simulink model "LKATestBenchExample"  (R2025b)
settings: Solver=VariableStepAuto  StartTime=0.0  StopTime=simStopTime  RelTol=1e-3
PostLoadFcn:
  | helperLKASetUp
StartFcn:
  | %sound(y_audio,Fs_audio);
values from neighbouring files (symbols this model uses):
  egoID = egoVehicle.ActorID    [helperLKASetUp.m]
  lr = 1.6    [helperLKASetUp.m]
  m = 1575    [helperLKASetUp.m]
  simStopTime = 30    [createDriverPath.m]
  Ts_3D = 0.1    [helperLKASetUp.m]
undefined symbols (not defined in the file or in its folder): Curvature, CurvatureDerivative, driving, gray, HeadingAngle, LateralOffset, Left, Right, Sim3dSensor, Strength, v0_ego, x0_ego, y0_ego, yaw0_ego
libraries: drivingscenarioandsensors x3, vrlib x1, sim3dcameralib x1, sim3dlib x1, sim3dautolib x1, dspvision x1, autolibshared x1
CloseFcn:
  | helperLKACleanUp
settings Model: SimulationMode=accelerator  Creator=The MathWorks, Inc.  LastModifiedBy=diogo
settings SolverCC: AlgebraicLoopSolver=TrustRegion
settings DataIOCC: ReturnWorkspaceOutputs=off
settings DebuggingCC: ParameterPrecisionLossMsg=none  UnconnectedInputMsg=warning  UnconnectedOutputMsg=warning  UnconnectedLineMsg=warning  ArithmeticOperatorsInVariantConditions=warning
settings HardwareCC: ProdLongLongMode=on
settings ModelReferenceCC: EnableRefExpFcnMdlSchedulingChecks=on
settings SFSimCC: SimUseLocalCustomCode=off
settings RTWCC: RTWUseLocalCustomCode=off  GPUComputeCapability=3.5  DLArmComputeVersion=19.05

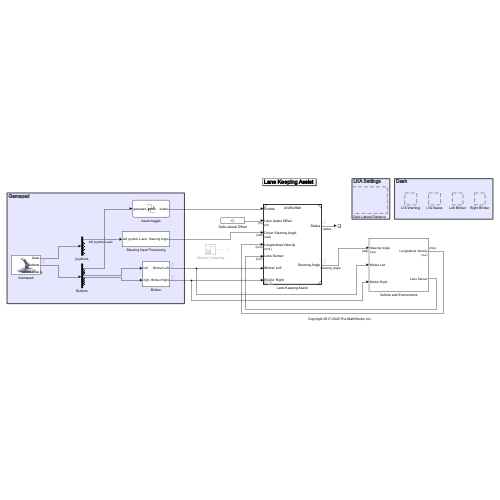
[thumbnail: Simulink's stored preview of the top-level diagram]
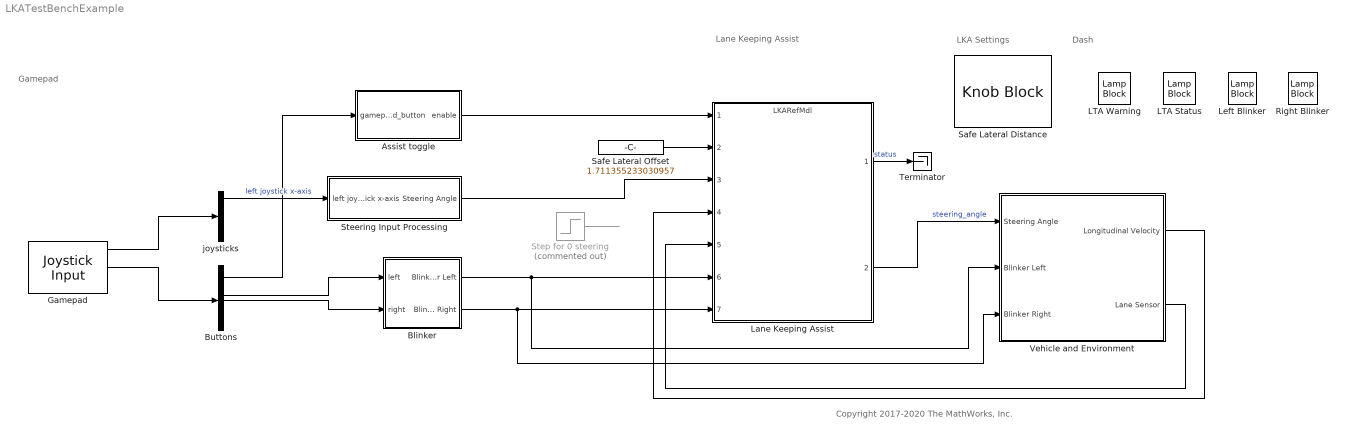
== system LKATestBenchExample ==
  note: Gamepad
  note: Lane Keeping Assist
  note: Copyright 2017-2020 The MathWorks, Inc.
  note: Dash
  note: LKA Settings
  Assist toggle : Stateflow chart  TreatAsAtomicUnit=on
  Blinker : Subsystem
  Buttons : Demux  Outputs=10
  Gamepad : vrlib/Joystick Input  joyid=1  adjustports=on  forcefeed=off
  LTA Status : LampBlock  LabelPosition=Hide  DefaultColor=[237.0, 177.0, 32.0]
  LTA Warning : LampBlock  LabelPosition=Hide  DefaultColor=[254.0, 51.0, 10.0]  Icon=StabilityControl
  Lane Keeping Assist : ModelReference  StartFcn=|  ModelNameDialog=LKARefMdl.slx  SimulationMode=Normal  CodeInterface=Top model  ModelReferenceVersion=11.20
      | load("helper_3d_model.mat");
      | sound(y_audio,Fs_audio)
  Left Blinker : LampBlock  LabelPosition=Hide  DefaultColor=[0.0, 0.0, 41.0]  Icon=TurnSignalLeft
  Right Blinker : LampBlock  LabelPosition=Hide  DefaultColor=[0.0, 0.0, 41.0]  Icon=TurnSignalRight
  Safe Lateral Distance : KnobBlock  LabelPosition=Hide  ScaleMax=2  TickInterval=0.5
  Safe Lateral Offset : Constant  Value=1.711355233030957  OutDataTypeStr=Inherit: Inherit via back propagation
  Steering Input Processing : Subsystem
  Step for 0 steering : Step  Commented=on  Time=simStopTime  After=0  OutDataTypeStr=Inherit: Inherit via back propagation  SampleTime=0
  Terminator : Terminator
  Vehicle and Environment : Subsystem
  joysticks : Demux  Outputs=5
  wires:
  Lane Keeping Assist/1 -> Terminator/1  "status"
  Lane Keeping Assist/2 -> Vehicle and Environment/1(Steering Angle)  "steering_angle"
  Vehicle and Environment/2(Lane Sensor) -> Lane Keeping Assist/5
  Safe Lateral Offset/1 -> Lane Keeping Assist/2
  Vehicle and Environment/1(Longitudinal Velocity) -> Lane Keeping Assist/4
  Gamepad/1 -> joysticks/1
  Step for 0 steering/1 -> ?
  Gamepad/2 -> Buttons/1
  Buttons/5 -> Blinker/1(left)
  Buttons/6 -> Blinker/2(right)
  Buttons/1 -> Assist toggle/1(gamepad_button)
  Assist toggle/1(enable) -> Lane Keeping Assist/1
  joysticks/1 -> Steering Input Processing/1(left joystick x-axis)  "left joystick x-axis"
  Steering Input Processing/1(Steering Angle) -> Lane Keeping Assist/3
  Blinker/2(Blinker Right) -> Vehicle and Environment/3(Blinker Right), Lane Keeping Assist/7
  Blinker/1(Blinker Left) -> Vehicle and Environment/2(Blinker Left), Lane Keeping Assist/6

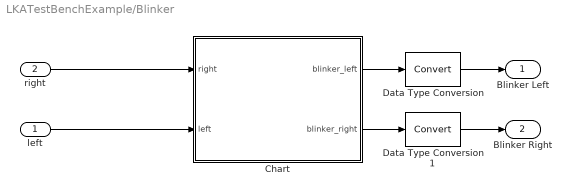
== system LKATestBenchExample/Blinker ==
  left : Inport
  right : Inport  Port=2
  Chart : Stateflow chart  TreatAsAtomicUnit=on
  Data Type Conversion : DataTypeConversion  SaturateOnIntegerOverflow=off  RndMeth=Floor
  Data Type Conversion1 : DataTypeConversion  SaturateOnIntegerOverflow=off  RndMeth=Floor
  Blinker Left : Outport
  Blinker Right : Outport  Port=2
  wires:
  right/1 -> Chart/1(right)
  Chart/1(blinker_left) -> Data Type Conversion/1
  Data Type Conversion/1 -> Blinker Left/1
  Data Type Conversion1/1 -> Blinker Right/1
  Chart/2(blinker_right) -> Data Type Conversion1/1
  left/1 -> Chart/2(left)

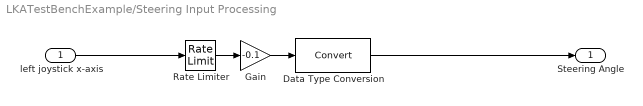
== system LKATestBenchExample/Steering Input Processing ==
  left joystick x-axis : Inport
  Data Type Conversion : DataTypeConversion  SaturateOnIntegerOverflow=off  RndMeth=Floor
  Gain : Gain  Gain=-0.1
  Rate Limiter : RateLimiter  SampleTimeMode=inherited
  Steering Angle : Outport
  wires:
  left joystick x-axis/1 -> Rate Limiter/1
  Gain/1 -> Data Type Conversion/1
  Data Type Conversion/1 -> Steering Angle/1
  Rate Limiter/1 -> Gain/1

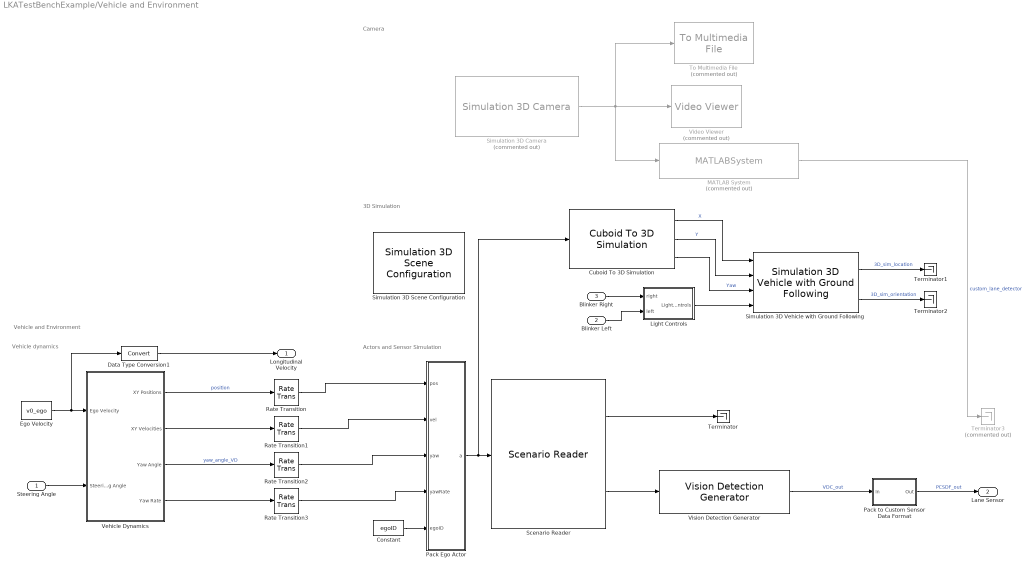
== system LKATestBenchExample/Vehicle and Environment ==
  note: Vehicle dynamics
  note: Camera
  note: Vehicle and Environment
  note: Actors and Sensor Simulation
  note: 3D Simulation
  Steering Angle : Inport  Unit=rad
  Blinker Left : Inport  Port=2
  Blinker Right : Inport  Port=3
  Constant : Constant  Value=egoID
  Cuboid To 3D Simulation : drivingscenarioandsensors/Cuboid To 3D Simulation  SpecifyActorID=off  ActorIDToConvert=1  SimulateUsing=Interpreted execution
  Data Type Conversion1 : DataTypeConversion  SaturateOnIntegerOverflow=off  RndMeth=Floor
  Ego Velocity : Constant  Value=v0_ego
  Light Controls : Subsystem
  MATLAB System : MATLABSystem  Commented=on  System=HelperLaneDetectorWrapper  EnableLaneTracker=on  EnableDisplays=on  Camera=struct('ImageSize',[480 640],'PrincipalPoint',[320 240],'FocalLength',[554 554],'Position',[0.57 0 1.45],'PositionSim3d',[0.57 0 1.45],'Rotation',[0 0 0],'LaneDetectionRanges',[6 30],'DetectionRanges',[6 50],'MeasurementNoise',diag([6,1,1]))  SimulateUsing=Code generation
      mask Type: HelperLaneDetectorWrapper
  Pack Ego Actor : MATLAB Function  TreatAsAtomicUnit=on
  Pack to Custom Sensor Data Format : Subsystem
  Rate Transition{,1..3} (4 alike) : RateTransition  OutPortSampleTime=Ts
  Scenario Reader : drivingscenarioandsensors/Scenario Reader  ScenarioSource=From workspace  ScenarioFileName=LKATestBenchScenario.mat  ScenarioVariableName=scenario  OutputCoordinateSystem=Vehicle coordinates  EgoVehicleSource=Input port  EgoVehicleActorID=egoID  OrientVehiclesOnRoad=off  OutputEgoVehiclePose=off  OutputEgoVehicleState=off  SampleTime=Ts_3D  LaneBoundaryOutput=Ego vehicle lane boundaries  LaneBoundaryDistance=0:0.5:60  LaneBoundaryLocation=Inner edge of lane markings  BusNameSource=Auto  BusName=BusActors  BusNumActorsSource=Scenario  BusNumActors=100  BusName2Source=Auto  BusName2=BusLaneBoundaries  BusNumLaneBoundariesSource=Scenario  BusNumLaneBoundaries=10  BusName3Source=Auto  BusName3=BusEgoActor  BusName4Source=Auto  BusName4=BusEgoState  ShowCoordinateLabels=on  SimulateUsing=Interpreted execution
  Simulation 3D Camera : sim3dcameralib/Simulation 3D Camera  Priority=1  Commented=on  sensorTag=Sim3dSensor�  sensorId=1  sensorName=Sim3dSensor�  vehTagList={'Scene Origin';'SimulinkVehicle1'}  vehTag=SimulinkVehicle1  CoordinateSystem=ISO8855  mountLoc=Roof center  offsetFlag=on  tmountOffset=[0.57 0 1.45]  extTmount=off  rmountOffset=[0, 0, 0]  extRmount=off  FocalLength=[554, 554]  OpticalCenter=[320, 240]  ImageSize=[480, 640]  RadialDistortion=[0, 0]  TangentialDistortion=[0, 0]  SensorSkew=0  VisualizeFieldOfView=off  FieldOfViewRange=61  DepthOutportEnabled=off  SemanticOutportEnabled=off  TransformOutportEnabled=off  SampleTime=Ts_3D  mountPoint=[0.57 0 1.45]  mountOrientation=[0 0 0]  aMode=3  ID=1
      settings: LibrarySourceBlock=drivingsim3d/Simulation 3D Camera
  Simulation 3D Scene Configuration : sim3dlib/Simulation 3D Scene Configuration  Priority=0  ProjectFormat=Default Scenes  SceneDesc=Curved road  ProjectName=C:\Program Files\MATLAB\R2025b\toolbox\shared\sim3d_projects\automotive_project_windows\UE\WindowsNoEditor\VehicleSimulation.exe  ScenePath=/Game/Maps/HwStrght  EnableOpenDRIVE=on  OpenDRIVEName=C:\Users\Miguel Fialho\Desktop\IST\MEEC\1º Ano\1º Semestre\Rob\Labs\Lab 1\Matlab\custom_road_2_export_V1.6.xodr  vehTagList={'Custom';'Scene Origin';'SimulinkVehicle1'}  vehTag=SimulinkVehicle1  AttachedCameraRelativeTranslation=[0 0 0]  FreeCameraDefaultInitialTranslation=[-6, 0, 2]  AttachedCameraRelativeRotation=[0 0 0]  FreeCameraDefaultInitialRotation=[0, -15, 0]  ViewpointName=Custom  FreeCameraInitialTranslation=[0, 0, 0]  ViewpointTranslation=[0 0 0]  FreeCameraInitialRotation=[0, 0, 0]  ViewpointRotation=[0 0 0]  OpVisEn=off  Ts=Ts_3D  EnableWindow=on  EnableRemoteAccess=off  EnableWeather=off  SunAzimuth=90  SunAltitude=40.0  EnableGeospatialSun=off  Latitude=0  Longitude=0  Date=2023-01-01  Time=10:30:00  GeoTimeZone=-5.0  SunDaylightSaving=off  wind=1  clouds=10  EnableVolumetricClouds=off  CloudCoverage=0  CloudAltitude=6  fog=0  rain=0  RaindropsEffect=off  SnowDensity=0  EnableGeospatial=off  TilesetSource=Earth terrain  UseTrueOrigin=off  OriginHeight=200  OriginLatitude=40.744652  OriginLongitude=-73.988864  MapStyle=Aerial  AdditionalAssetIDs=[]  UseAdvancedSunSky=off  SolarTime=11  TimeZone=-5  Day=21  Month=9  Year=2022  UseDaylightSavingTime=on  DSTStartDay=10  DSTStartMonth=3  DSTEndDay=3  DSTEndMonth=11  DSTSwitchHour=2  sensorTag=MainCamera1  sensorId=1  sensorName=MainCamera1  mountLoc=Origin  offsetFlag=off  tmountOffset=[0, 0, 0]  rmountOffset=[0, 0, 0]  HorizontalResolution=1280  VerticalResolution=720  HorizontalFOV=60  mountPoint=[0 0 0]  mountOrientation=[0 0 0]  aMode=5  ID=1  GeoTrigger=Inactive  ViewNameList={'Custom'}  ViewTranslationList={'[0 0 0]'}  ViewRotationList={'[0 0 0]'}
      settings: LibrarySourceBlock=sl3dlib/Simulation 3D/Environment/Simulation 3D Scene Configuration
  Simulation 3D Vehicle with Ground Following : sim3dautolib/Simulation 3D Vehicle with Ground Following  Priority=-1  PassVehMesh=Muscle car  MeshPath=/MathWorksAutomotiveContent/Vehicles/Muscle/Meshes/SK_MuscleCar.SK_MuscleCar  TrackWidth=1.9  WheelBase=3  WheelRadius=0.35  VehColor=Red  CoordinateSystem=ISO8855  InitialPos=[0, 0, 0]  InitialRot=[0, 0, 0]  ActorName=SimulinkVehicle1  SampleTime=Ts_3D  ActorType=SimulinkVehicle  ID=1  aMode=3  ActorTag=SimulinkVehicle1  CoordinateScheme=0  VehLightsControl=on  HeadlightColor=[ 1, 1, 1 ]  HighBeamIntensity=100000  LowBeamIntensity=60000  HighBeamConeAngle=70  LowBeamConeAngle=70  LeftHeadlightOrientation=[ 0, 0 ]  RightHeadlightOrientation=[ 0, 0 ]  BrakelightIntensity=500  ReverselightIntensity=500  SignallightIntensity=500  SignallightPeriod=1  SignalPulseWidth=50  TransformOutportEnabled=on
      settings: LibrarySourceBlock=drivingsim3d/Simulation 3D Vehicle with Ground Following
  Terminator : Terminator
  Terminator1 : Terminator
  Terminator2 : Terminator
  Terminator3 : Terminator  Commented=on
  To Multimedia File : dspvision/To Multimedia File  Commented=on  outputFilename=C:\Users\Miguel Fialho\Documents\MATLAB\Examples\R2025b\autonomous_control\LaneKeepingAssistWithLaneDetectionExample\output.mp4  streamSelection=Video only  videoCompressor=None (uncompressed)  audioCompressor=None (uncompressed)  imagePorts=One multidimensional signal  fileType=MPEG4  audioDatatype=Determine from input data type  fourcc=RGB  audioBitRate=128  audioQuality=75  videoQuality=75  mj2000CompFactor=10
      settings: LibrarySourceBlock=visionsinks/To Multimedia File
  Vehicle Dynamics : Subsystem  VariantControl=VariantVDBS
  Video Viewer : VideoViewer  Commented=on  colormapValue=gray(256)  FigPos=[1 814 1536 717]
  Vision Detection Generator : drivingscenarioandsensors/Vision Detection Generator  SensorIndex=1  DetectorOutput=Lanes only  UpdateInterval=Ts  LaneUpdateInterval=Ts  SensorLocation=[ 1.9, 0 ]  Height=1.1  Yaw=0  Pitch=1  Roll=0  BusNameSource=Auto  BusName=BusObjectDetections  BusName2Source=Property  BusName2=BusVision  MaxNumDetectionsSource=Property  MaxNumDetections=50  MaxNumLanesSource=Property  MaxNumLanes=2  DetectionCoordinates=Ego Cartesian  SimulateUsing=Interpreted execution  MaxRange=150  BoundingBoxAccuracy=5  ProcessNoiseIntensity=5  MaxSpeed=50  MaxAllowedOcclusion=0.5  MinObjectImageSize=[ 15, 15 ]  DetectionProbability=0.9  FalsePositivesPerImage=0.1  MinLaneImageSize=[ 20, 3 ]  LaneBoundaryAccuracy=3  HasNoise=on  InitialSeedSource=Repeatable  InitialSeed=0  UsedSeed=driving.internal.SimulinkUtilities.seedManager(gcb)  ActorProfilesSource=Parameters  ActorProfilesParameters=driving.internal.ActorProfilesParameters  ActorProfilesExpression=struct( 'ClassID', 0, 'Length', 4.7, 'Width', 1.8, 'Height', 1.4, 'OriginOffset', [ -1.35, 0, 0 ] )  Intrinsics=driving.internal.cameraIntrinsics
  Longitudinal Velocity : Outport  OutDataTypeStr=single  Unit=m/s  VectorParamsAs1DForOutWhenUnconnected=off
  Lane Sensor : Outport  Port=2  VectorParamsAs1DForOutWhenUnconnected=off
  wires:
  Ego Velocity/1 -> Data Type Conversion1/1, Vehicle Dynamics/1(Ego Velocity)
  Scenario Reader/1 -> Terminator/1
  Pack Ego Actor/1(a) -> Cuboid To 3D Simulation/1, Scenario Reader/1
  Vehicle Dynamics/2(XY Velocities) -> Rate Transition1/1
  Vehicle Dynamics/3(Yaw Angle) -> Rate Transition2/1  "yaw_angle_VD"
  Rate Transition/1 -> Pack Ego Actor/1(pos)
  Vehicle Dynamics/4(Yaw Rate) -> Rate Transition3/1
  Rate Transition2/1 -> Pack Ego Actor/3(yaw)
  Rate Transition1/1 -> Pack Ego Actor/2(vel)
  Rate Transition3/1 -> Pack Ego Actor/4(yawRate)
  Scenario Reader/2 -> Vision Detection Generator/1
  Vehicle Dynamics/1(XY Positions) -> Rate Transition/1  "position"
  Steering Angle/1 -> Vehicle Dynamics/2(Steering Angle)
  Vision Detection Generator/1 -> Pack to Custom Sensor Data Format/1(In)  "VDC_out"
  Pack to Custom Sensor Data Format/1(Out) -> Lane Sensor/1  "PCSDF_out"
  Data Type Conversion1/1 -> Longitudinal Velocity/1
  Constant/1 -> Pack Ego Actor/5(egoID)
  Cuboid To 3D Simulation/1 -> Simulation 3D Vehicle with Ground Following/1  "X"
  Cuboid To 3D Simulation/2 -> Simulation 3D Vehicle with Ground Following/2  "Y"
  Cuboid To 3D Simulation/3 -> Simulation 3D Vehicle with Ground Following/3  "Yaw"
  Simulation 3D Vehicle with Ground Following/1 -> Terminator1/1  "3D_sim_location"
  Simulation 3D Vehicle with Ground Following/2 -> Terminator2/1  "3D_sim_orientation"
  Simulation 3D Camera/1 -> MATLAB System/1, To Multimedia File/1, Video Viewer/1
  MATLAB System/1 -> Terminator3/1  "custom_lane_detector"
  Blinker Right/1 -> Light Controls/1(right)
  Blinker Left/1 -> Light Controls/2(left)
  Light Controls/1(Light Controls) -> Simulation 3D Vehicle with Ground Following/4

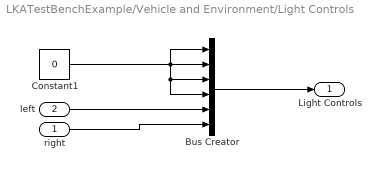
== system LKATestBenchExample/Vehicle and Environment/Light Controls ==
  right : Inport
  left : Inport  Port=2
  Bus Creator : BusCreator  Inputs=6
  Constant1 : Constant  Value=0  OutDataTypeStr=boolean
  Light Controls : Outport
  wires:
  Constant1/1 -> Bus Creator/4, Bus Creator/3, Bus Creator/1, Bus Creator/2
  right/1 -> Bus Creator/6
  Bus Creator/1 -> Light Controls/1
  left/1 -> Bus Creator/5

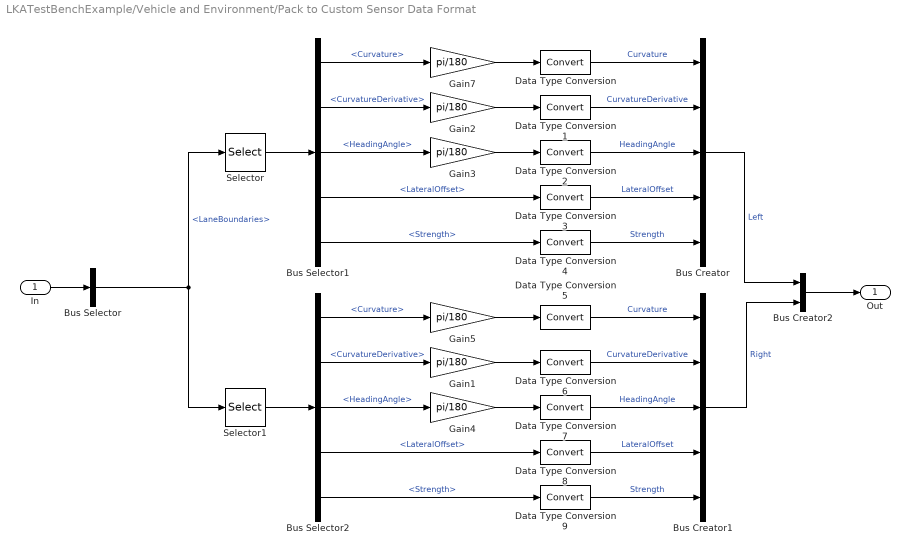
== system LKATestBenchExample/Vehicle and Environment/Pack to Custom Sensor Data Format ==
  In : Inport
  Bus Creator : BusCreator  Inputs=Curvature,CurvatureDerivative,HeadingAngle,LateralOffset,Strength  OutDataTypeStr=Bus: LaneSensorBoundaries
  Bus Creator1 : BusCreator  Inputs=Curvature,CurvatureDerivative,HeadingAngle,LateralOffset,Strength  OutDataTypeStr=Bus: LaneSensorBoundaries
  Bus Creator2 : BusCreator  Inputs=Left,Right  OutDataTypeStr=Bus: LaneSensor
  Bus Selector : BusSelector  OutputSignals=LaneBoundaries
  Bus Selector1 : BusSelector  OutputSignals=Curvature,CurvatureDerivative,HeadingAngle,LateralOffset,Strength
  Bus Selector2 : BusSelector  OutputSignals=Curvature,CurvatureDerivative,HeadingAngle,LateralOffset,Strength
  Data Type Conversion{,1..9} (10 alike) : DataTypeConversion  SaturateOnIntegerOverflow=off  RndMeth=Floor
  Gain{1..5,7} (6 alike) : Gain  Gain=pi/180
  Selector : Selector  InputPortWidth=2  IndexOptions=Index vector (dialog)  Indices=1  OutputSizes=1
  Selector1 : Selector  InputPortWidth=2  IndexOptions=Index vector (dialog)  Indices=2  OutputSizes=1
  Out : Outport  VectorParamsAs1DForOutWhenUnconnected=off
  wires:
  In/1 -> Bus Selector/1
  Bus Selector/1 -> Selector/1, Selector1/1  "<LaneBoundaries>"
  Selector/1 -> Bus Selector1/1
  Bus Selector1/2 -> Gain2/1  "<CurvatureDerivative>"
  Bus Selector1/1 -> Gain7/1  "<Curvature>"
  Bus Selector1/3 -> Gain3/1  "<HeadingAngle>"
  Gain7/1 -> Data Type Conversion/1
  Gain2/1 -> Data Type Conversion1/1
  Gain3/1 -> Data Type Conversion2/1
  Bus Selector1/4 -> Data Type Conversion3/1  "<LateralOffset>"
  Bus Selector1/5 -> Data Type Conversion4/1  "<Strength>"
  Data Type Conversion/1 -> Bus Creator/1  "Curvature"
  Data Type Conversion1/1 -> Bus Creator/2  "CurvatureDerivative"
  Data Type Conversion2/1 -> Bus Creator/3  "HeadingAngle"
  Data Type Conversion3/1 -> Bus Creator/4  "LateralOffset"
  Data Type Conversion4/1 -> Bus Creator/5  "Strength"
  Data Type Conversion9/1 -> Bus Creator1/5  "Strength"
  Data Type Conversion6/1 -> Bus Creator1/2  "CurvatureDerivative"
  Data Type Conversion7/1 -> Bus Creator1/3  "HeadingAngle"
  Data Type Conversion8/1 -> Bus Creator1/4  "LateralOffset"
  Data Type Conversion5/1 -> Bus Creator1/1  "Curvature"
  Bus Selector2/1 -> Gain5/1  "<Curvature>"
  Selector1/1 -> Bus Selector2/1
  Bus Selector2/4 -> Data Type Conversion8/1  "<LateralOffset>"
  Bus Selector2/5 -> Data Type Conversion9/1  "<Strength>"
  Bus Selector2/2 -> Gain1/1  "<CurvatureDerivative>"
  Gain4/1 -> Data Type Conversion7/1
  Gain5/1 -> Data Type Conversion5/1
  Gain1/1 -> Data Type Conversion6/1
  Bus Selector2/3 -> Gain4/1  "<HeadingAngle>"
  Bus Creator2/1 -> Out/1
  Bus Creator/1 -> Bus Creator2/1  "Left"
  Bus Creator1/1 -> Bus Creator2/2  "Right"

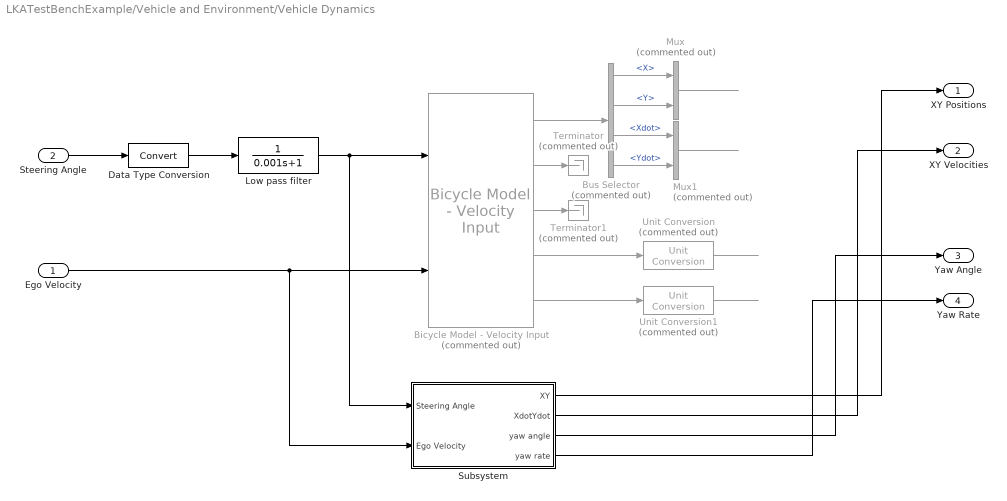
== system LKATestBenchExample/Vehicle and Environment/Vehicle Dynamics ==
  Ego Velocity : Inport
  Steering Angle : Inport  Port=2
  Bicycle Model - Velocity Input : autolibshared/Bicycle Model - Velocity Input  Commented=on  trackMode=Single (bicycle)  inputMode=External longitudinal forces  frontSteerMode=on  rearSteerMode=off  windMode=off  muMode=off  extFMode=off  extMMode=off  aMode=3  NF=2  NR=2  m=m  a=lf  b=lr  h=0.35  X_o=x0_ego  xdot_o=0  CalphaMode=off  sigmaMode=on  w=[1.4,1.4]  Cy_f=Cf  Cy_r=Cr  sigma_f=.1  sigma_r=.1  alpha_f_brk=[-.1 .1]  Cy_f_data=[-9e3 9e3]  alpha_r_brk=[-.1 .1]  Cy_r_data=[-9e3 9e3]  Y_o=y0_ego  ydot_o=0  Izz=Iz  psi_o=yaw0_ego*pi/180  r_o=0  Af=2  Cd=.3  Cl=.1  Cpm=.1  beta_w=[0:0.01:0.3]  Cs=[0:0.03:0.9]  Cym=[0:0.01:0.3]  Pabs=101325  Tair=273  g=9.81  mu=1  xdot_tol=.01  Fznom=5000  Fxtire_sat=1e6  Fytire_sat=1e6  longOff=0  latOff=0  vertOff=0
      settings: LibrarySourceBlock=drivingscenarioandsensors/Bicycle Model - Velocity Input
  Bus Selector : BusSelector  Commented=on  OutputSignals=InertFrm.FrntAxl.Disp.X,InertFrm.FrntAxl.Disp.Y,InertFrm.FrntAxl.Vel.Xdot,InertFrm.FrntAxl.Vel.Ydot
  Data Type Conversion : DataTypeConversion  SaturateOnIntegerOverflow=off  RndMeth=Floor
  Low pass filter : TransferFcn  Denominator=[0.001 1]
  Mux : Mux  Commented=on  Inputs=2
  Mux1 : Mux  Commented=on  Inputs=2
  Subsystem : Subsystem
  Terminator : Terminator  Commented=on
  Terminator1 : Terminator  Commented=on
  Unit Conversion : UnitConversion  Commented=on  OutputType=Inherit: Inherit via back propagation
  Unit Conversion1 : UnitConversion  Commented=on  OutputType=Inherit: Inherit via back propagation
  XY Positions : Outport  Unit=m  VectorParamsAs1DForOutWhenUnconnected=off
  XY Velocities : Outport  Port=2  Unit=m/s  VectorParamsAs1DForOutWhenUnconnected=off
  Yaw Angle : Outport  Port=3  Unit=deg  VectorParamsAs1DForOutWhenUnconnected=off
  Yaw Rate : Outport  Port=4  Unit=degree/s  VectorParamsAs1DForOutWhenUnconnected=off
  wires:
  Unit Conversion1/1 -> ?
  Ego Velocity/1 -> Subsystem/2(Ego Velocity), Bicycle Model - Velocity Input/2
  Bicycle Model - Velocity Input/1 -> Bus Selector/1
  Bicycle Model - Velocity Input/2 -> Terminator/1
  Bicycle Model - Velocity Input/3 -> Terminator1/1
  Bicycle Model - Velocity Input/4 -> Unit Conversion/1
  Bicycle Model - Velocity Input/5 -> Unit Conversion1/1
  Bus Selector/1 -> Mux/1  "<X>"
  Bus Selector/2 -> Mux/2  "<Y>"
  Bus Selector/3 -> Mux1/1  "<Xdot>"
  Bus Selector/4 -> Mux1/2  "<Ydot>"
  Data Type Conversion/1 -> Low pass filter/1
  Steering Angle/1 -> Data Type Conversion/1
  Low pass filter/1 -> Subsystem/1(Steering Angle), Bicycle Model - Velocity Input/1
  Subsystem/1(XY) -> XY Positions/1
  Subsystem/2(XdotYdot) -> XY Velocities/1
  Subsystem/3(yaw angle) -> Yaw Angle/1
  Subsystem/4(yaw rate) -> Yaw Rate/1
  Mux1/1 -> ?
  Unit Conversion/1 -> ?
  Mux/1 -> ?

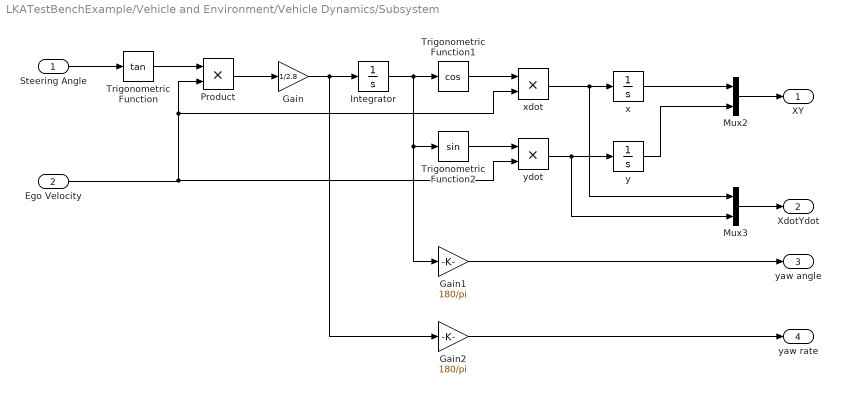
== system LKATestBenchExample/Vehicle and Environment/Vehicle Dynamics/Subsystem ==
  Steering Angle : Inport
  Ego Velocity : Inport  Port=2
  Gain : Gain  Gain=1/2.8
  Gain1 : Gain  Gain=180/pi
  Gain2 : Gain  Gain=180/pi
  Integrator : Integrator  InitialCondition=yaw0_ego*(pi/180)
  Mux2 : Mux  Inputs=2
  Mux3 : Mux  Inputs=2
  Product : Product
  Trigonometric Function : Trigonometry  Operator=tan
  Trigonometric Function1 : Trigonometry  Operator=cos
  Trigonometric Function2 : Trigonometry
  x : Integrator  InitialCondition=x0_ego
  xdot : Product
  y : Integrator  InitialCondition=y0_ego
  ydot : Product
  XY : Outport
  XdotYdot : Outport  Port=2
  yaw angle : Outport  Port=3
  yaw rate : Outport  Port=4
  wires:
  Trigonometric Function2/1 -> ydot/1
  ydot/1 -> y/1, Mux3/2
  Trigonometric Function/1 -> Product/1
  x/1 -> Mux2/1
  xdot/1 -> x/1, Mux3/1
  Trigonometric Function1/1 -> xdot/1
  Integrator/1 -> Gain1/1, Trigonometric Function2/1, Trigonometric Function1/1
  Product/1 -> Gain/1
  Mux2/1 -> XY/1
  Gain/1 -> Gain2/1, Integrator/1
  y/1 -> Mux2/2
  Ego Velocity/1 -> ydot/2, Product/2, xdot/2
  Steering Angle/1 -> Trigonometric Function/1
  Gain2/1 -> yaw rate/1
  Gain1/1 -> yaw angle/1
  Mux3/1 -> XdotYdot/1

== stateflow chart LKATestBenchExample/Assist toggle ==
  state Off
    entry:
    enable = false;
  state On
    entry:
    enable = true;
  (default) -> On
  Off -> On : [gamepad_button == 1 && after(0.5, sec)]
  On -> Off : [gamepad_button == 1 && after(0.5, sec)]
  data: gamepad_button input; enable output boolean

== stateflow chart LKATestBenchExample/Blinker/Chart ==
  state Off
    entry:
    blinker_right = 0;
    blinker_left = 0;
  state Left
    entry:
    blinker_left = 1;
    blinker_right = 0;
  state Right
    entry:
    blinker_right = 1;
    blinker_left = 0;
  (default) -> Off
  Off -> Left [order 1] : [left == 1 && after(0.5, sec)]
  Left -> Off [order 2] : [left == 1 && after(0.5, sec)]
  Right -> Off [order 2] : [right == 1 && after(0.5, sec)]
  Off -> Right [order 2] : [right == 1 && after(0.5, sec)]
  Right -> Left [order 1] : [left == 1 && after(0.5, sec)]
  Left -> Right [order 1] : [right == 1 && after(0.5, sec)]
  data: right input; blinker_left output; blinker_right output; left input

== matlab function LKATestBenchExample/Vehicle and Environment/Pack Ego Actor ==
  data: pos input; a output Bus: BusActor size=1; vel input; yaw input; yawRate input; egoID input
function a = packEgo(pos,vel,yaw,yawRate,egoID)
% Pack ego information into a single ego actor bus
%
% Imoprtant note:
% Output is a bus of type BusActorsActors. This is the same bus used by the
% Scenario Reader to output an individual actor. If you change the
% output bus name of Scenario Reader change the output bus name here
% as well by clicking on 'Edit Data' in the menu above.

a = struct(...
    'ActorID',egoID,...
    'Position', [pos(1) pos(2) 0], ...
    'Velocity', [vel(1) vel(2) 0], ...
    'Roll', 0, ...
    'Pitch', 0, ...
    'Yaw', yaw, ...
    'AngularVelocity', [0 0 yawRate]);
